simulink library "INT_ASDrf_Governor"  (R2016b)
settings: Solver=VariableStepAuto  StartTime=0.0  StopTime=10.0  RelTol=1e-3
settings Model: Creator=lenovo  LastModifiedBy=lenovo

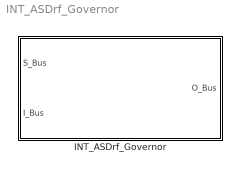
== system INT_ASDrf_Governor ==
  INT_ASDrf_Governor : Subsystem

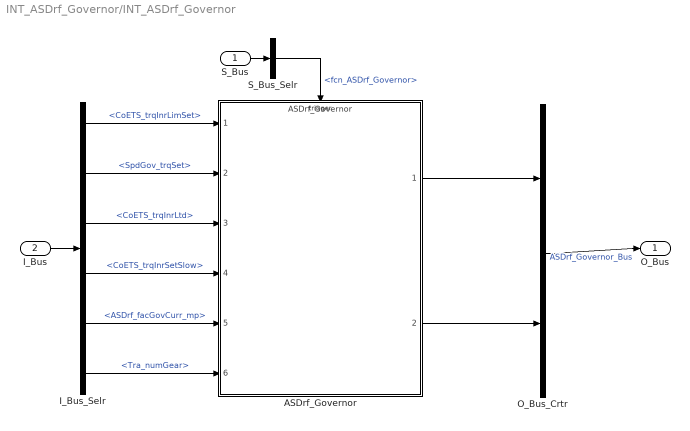
== system INT_ASDrf_Governor/INT_ASDrf_Governor ==
  S_Bus : Inport
  I_Bus : Inport  Port=2
  ASDrf_Governor : ModelReference  ModelNameDialog=ASDrf_Governor  SimulationMode=Normal  ModelReferenceVersion=1.10  TriggerPortName=function  TriggerPortTriggerType=function-call  TriggerPortStatesWhenEnabling=held
  I_Bus_Selr : BusSelector  OutputSignals=CoETS_trqInrLimSet,SpdGov_trqSet,CoETS_trqInrLtd,CoETS_trqInrSetSlow,ASDrf_facGovCurr_mp,Tra_numGear
  O_Bus_Crtr : BusCreator  Inputs=2
  S_Bus_Selr : BusSelector  OutputSignals=fcn_ASDrf_Governor
  O_Bus : Outport
  wires:
  S_Bus_Selr/1 -> ASDrf_Governor/Trigger  "<fcn_ASDrf_Governor>"
  S_Bus/1 -> S_Bus_Selr/1
  I_Bus/1 -> I_Bus_Selr/1
  I_Bus_Selr/1 -> ASDrf_Governor/1  "<CoETS_trqInrLimSet>"
  I_Bus_Selr/2 -> ASDrf_Governor/2  "<SpdGov_trqSet>"
  I_Bus_Selr/3 -> ASDrf_Governor/3  "<CoETS_trqInrLtd>"
  I_Bus_Selr/4 -> ASDrf_Governor/4  "<CoETS_trqInrSetSlow>"
  I_Bus_Selr/5 -> ASDrf_Governor/5  "<ASDrf_facGovCurr_mp>"
  I_Bus_Selr/6 -> ASDrf_Governor/6  "<Tra_numGear>"
  O_Bus_Crtr/1 -> O_Bus/1  "ASDrf_Governor_Bus"
  ASDrf_Governor/1 -> O_Bus_Crtr/1
  ASDrf_Governor/2 -> O_Bus_Crtr/2
